simulink model "BMSInputs"  (R2024b)
settings: Solver=FixedStepAuto  StartTime=0.0  StopTime=10.0  RelTol=1e-3  EnableMultiTasking=on
settings Model: DataDictionary=Master_Dictionary.sldd  EnableAccessToBaseWorkspace=off  Creator=torni  LastModifiedBy=Will
settings OptimizationCC: DefaultParameterBehavior=Inlined  EnhancedBackFolding=on  PassReuseOutputArgsAs=Individual arguments  ZeroExternalMemoryAtStartup=off  ZeroInternalMemoryAtStartup=off  MaxStackSize=8192  OptimizeBlockOrder=speed  DifferentSizesBufferReuse=on  OptimizationCustomize=off  EfficientTunableParamExpr=on
settings DebuggingCC: ParameterTunabilityLossMsg=error
settings HardwareCC: ProdBitPerPointer=32  ProdBitPerSizeT=32  ProdBitPerPtrDiffT=32  ProdLargestAtomicInteger=Long  ProdLargestAtomicFloat=Double  ProdWordSize=32  ProdLongLongMode=on  ProdHWDeviceType=ARM Compatible->ARM Cortex-M
settings SFSimCC: MATLABDynamicMemAlloc=off
settings RTWCC: Description=Embedded Coder  SystemTargetFile=ert.tlc  HardwareBoard=STM32H7xx Based (Single-core)  TemplateMakefile=ert_default_tmf  Toolchain=GNU Tools for ARM Embedded Processors
settings CodeAppCC: ForceParamTrailComments=on  IgnoreCustomStorageClasses=off  OperatorAnnotations=on  SimulinkDataObjDesc=on  SFDataObjDesc=on  InsertBlockDesc=on
settings ERTTargetCC: TargetLangStandard=C99 (ISO)  CodeReplacementLibrary=ARM Cortex-M  ExtModeTransport=3  ExtModeStaticAlloc=on  ExtModeStaticAllocSize=2048  ExtModeMexFile=ext_xcp  ExtModeIntrfLevel=Level2 - Open

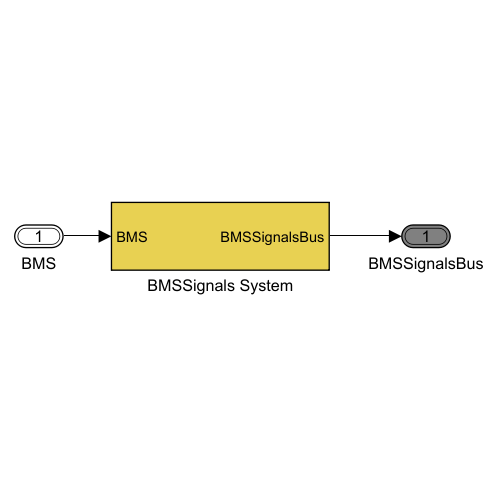
[thumbnail: Simulink's stored preview of the top-level diagram]
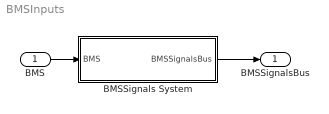
== system BMSInputs ==
  BMS : Inport  OutDataTypeStr=Bus: BMS
  BMSSignals System : Subsystem
  BMSSignalsBus : Outport  OutDataTypeStr=Bus: BMSSignals  VectorParamsAs1DForOutWhenUnconnected=off
  wires:
  BMS/1 -> BMSSignals System/1(BMS)
  BMSSignals System/1(BMSSignalsBus) -> BMSSignalsBus/1

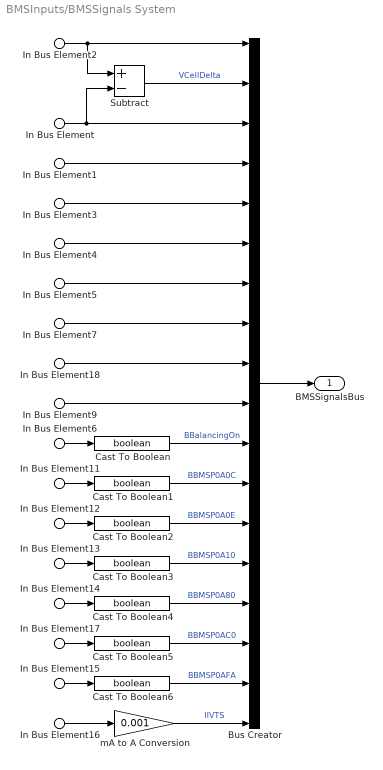
== system BMSInputs/BMSSignals System ==
  In Bus Element : Inport  PortName=BMS  Element=VCellMin
  In Bus Element1 : Inport  PortName=BMS  Element=VCellAverage
  In Bus Element2 : Inport  PortName=BMS  Element=VCellMax
  In Bus Element3 : Inport  PortName=BMS  Element=TCellMax
  In Bus Element5 : Inport  PortName=BMS  Element=TCellMin
  In Bus Element7 : Inport  PortName=BMS  Element=IBMSHallEffect
  In Bus Element9 : Inport  PortName=BMS  Element=RCellAverage
  In Bus Element11 : Inport  PortName=BMS  Element=BBMSP0A0C
  In Bus Element12 : Inport  PortName=BMS  Element=BBMSP0A0E
  In Bus Element13 : Inport  PortName=BMS  Element=BBMSP0A10
  In Bus Element14 : Inport  PortName=BMS  Element=BBMSP0A80
  In Bus Element15 : Inport  PortName=BMS  Element=BBMSP0AFA
  In Bus Element16 : Inport  PortName=BMS  Element=IIVTS
  In Bus Element17 : Inport  PortName=BMS  Element=BBMSP0AC0
  In Bus Element18 : Inport  PortName=BMS  Element=VDCAccumulator
  In Bus Element6 : Inport  PortName=BMS  Element=BBalancingOn
  In Bus Element4 : Inport  PortName=BMS  Element=IBMSDLC
  Bus Creator : BusCreator  Inputs=18  OutDataTypeStr=Bus: BMSSignals
  Cast To Boolean{,1..6} (7 alike) : DataTypeConversion  OutDataTypeStr=boolean  SaturateOnIntegerOverflow=off  RndMeth=Floor
  Subtract : Sum  Inputs=+-
  mA to A Conversion : Gain  Gain=0.001
  BMSSignalsBus : Outport  OutDataTypeStr=Bus: BMSSignals  VectorParamsAs1DForOutWhenUnconnected=off
  wires:
  Bus Creator/1 -> BMSSignalsBus/1
  In Bus Element/1 -> Bus Creator/3, Subtract/2
  In Bus Element1/1 -> Bus Creator/4
  In Bus Element2/1 -> Bus Creator/1, Subtract/1
  In Bus Element3/1 -> Bus Creator/5
  In Bus Element4/1 -> Bus Creator/6
  In Bus Element5/1 -> Bus Creator/7
  In Bus Element7/1 -> Bus Creator/8
  In Bus Element18/1 -> Bus Creator/9
  In Bus Element9/1 -> Bus Creator/10
  In Bus Element6/1 -> Cast To Boolean/1
  In Bus Element11/1 -> Cast To Boolean1/1
  In Bus Element12/1 -> Cast To Boolean2/1
  In Bus Element13/1 -> Cast To Boolean3/1
  In Bus Element14/1 -> Cast To Boolean4/1
  In Bus Element16/1 -> mA to A Conversion/1
  In Bus Element17/1 -> Cast To Boolean5/1
  Subtract/1 -> Bus Creator/2  "VCellDelta"
  mA to A Conversion/1 -> Bus Creator/18  "IIVTS"
  In Bus Element15/1 -> Cast To Boolean6/1
  Cast To Boolean/1 -> Bus Creator/11  "BBalancingOn"
  Cast To Boolean1/1 -> Bus Creator/12  "BBMSP0A0C"
  Cast To Boolean2/1 -> Bus Creator/13  "BBMSP0A0E"
  Cast To Boolean3/1 -> Bus Creator/14  "BBMSP0A10"
  Cast To Boolean4/1 -> Bus Creator/15  "BBMSP0A80"
  Cast To Boolean5/1 -> Bus Creator/16  "BBMSP0AC0"
  Cast To Boolean6/1 -> Bus Creator/17  "BBMSP0AFA"
